simulink model "Lab4_modello_simulink"  (R2024b)
settings: Solver=VariableStepAuto  StartTime=0.0  StopTime=10  MaxStep=1e-3  RelTol=1e-3
values from neighbouring files (symbols this model uses):
  A = [0 1; (2*Km*(Im)^2)/(m*(x1)^3) 0]    [Lab4.m]
  alfa = 1/(dcgain(H_pippo))    [Lab4.m]
  B = [0 -(2*Km*Im)/(m*(x1)^2)]'    [Lab4.m]
  C = [Kt 0]    [Lab4.m]
  g = 9.81    [Lab4.m]    (also in generate_levitator.m)
  Im = 0.8    [Lab4.m]
  K = place(A,B,autoval)    [Lab4.m]
  Km = 1.52e-4    (= 0.000152)    [Lab4.m]    (also in generate_levitator.m)
  Kt = 708.27    [Lab4.m]    (also in generate_levitator.m)
  m = 0.02    [Lab4.m]    (also in generate_levitator.m)
undefined symbols (not defined in the file or in its folder): L, x1_eq
settings Model: Creator=stefa  LastModifiedBy=stefa

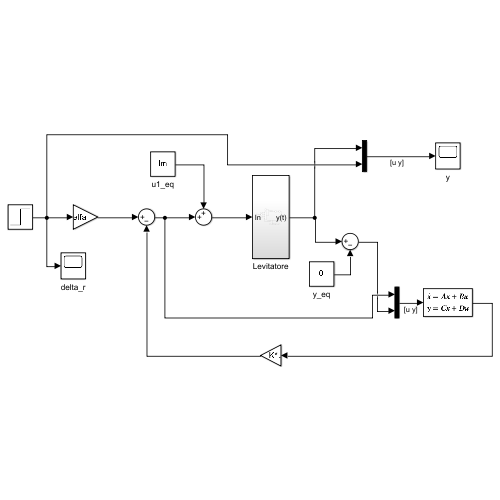
[thumbnail: Simulink's stored preview of the top-level diagram]
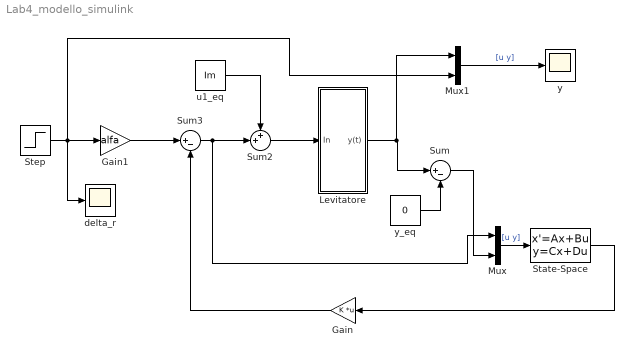
== system Lab4_modello_simulink ==
  Gain : Gain  Gain=K  Multiplication=Matrix(K*u)
  Gain1 : Gain  Gain=alfa
  Levitatore : Subsystem
  Mux : Mux  Inputs=2
  Mux1 : Mux  Inputs=2
  State-Space : StateSpace  A=A-L*C  B=[B L]  C=eye(2,2)  D=zeros(2,2)  InitialCondition=0
  Step : Step  Time=0  After=7  SampleTime=0
  Sum : Sum  Inputs=|+-
  Sum2 : Sum  Inputs=++|
  Sum3 : Sum  Inputs=|+-
  delta_r : Scope
  u1_eq : Constant  Value=Im
  y : Scope
  y_eq : Constant  Value=0
  wires:
  y_eq/1 -> Sum/2
  Sum2/1 -> Levitatore/1(In)
  Gain/1 -> Sum3/2
  u1_eq/1 -> Sum2/1
  Sum3/1 -> Mux/1, Sum2/2
  Gain1/1 -> Sum3/1
  Step/1 -> Gain1/1, Mux1/2, delta_r/1
  State-Space/1 -> Gain/1
  Levitatore/1(y(t)) -> Mux1/1, Sum/1
  Mux/1 -> State-Space/1  "[u y]"
  Mux1/1 -> y/1  "[u y]"
  Sum/1 -> Mux/2

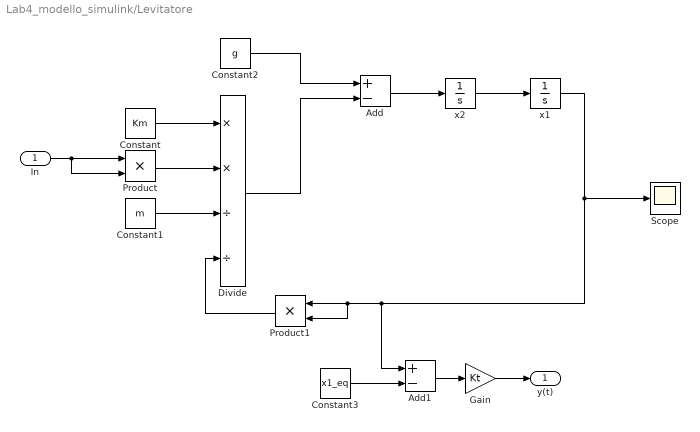
== system Lab4_modello_simulink/Levitatore ==
  In : Inport
  Add : Sum  Inputs=+-
  Add1 : Sum  Inputs=+-
  Constant : Constant  Value=Km
  Constant1 : Constant  Value=m
  Constant2 : Constant  Value=g
  Constant3 : Constant  Value=x1_eq
  Divide : Product  Inputs=**//
  Gain : Gain  Gain=Kt
  Product : Product
  Product1 : Product
  Scope : Scope
  x1 : Integrator  InitialCondition=x1_eq
  x2 : Integrator
  y(t) : Outport
  wires:
  Constant/1 -> Divide/1
  Constant1/1 -> Divide/3
  Product/1 -> Divide/2
  In/1 -> Product/2, Product/1
  Constant2/1 -> Add/1
  Divide/1 -> Add/2
  Add/1 -> x2/1
  x2/1 -> x1/1
  x1/1 -> Scope/1, Product1/2, Product1/1, Add1/1
  Product1/1 -> Divide/4
  Add1/1 -> Gain/1
  Gain/1 -> y(t)/1
  Constant3/1 -> Add1/2
